simulink model "BSCU_Brake_cmd_tmp"  (Simulink 8.4)
settings: Solver=ode45  StartTime=0.0  StopTime=10.0  RelTol=1e-3
undefined symbols (not defined in the file): BRAKE_PRESSURE_LO, BRAKE_PRESSURE_MAX, BRAKE_PRESSURE_MED, LO, MANUAL, MAX, MED
settings Model: Creator=bourbouh  LastModifiedBy=hbourbou  CovSFcnEnable=on
settings DataIOCC: LimitDataPoints=off  SaveFormat=StructureWithTime  SignalLoggingSaveFormat=Dataset
settings OptimizationCC: ExpressionDepthLimit=128
settings DebuggingCC: UnderspecifiedInitializationDetection=Simplified  MergeDetectMultiDrivingBlocksExec=error  SolverPrmCheckMsg=none  FcnCallInpInsideContextMsg=EnableAllAsError  FrameProcessingCompatibilityMsg=error  StateNameClashWarn=none
settings HardwareCC: ProdBitPerPointer=64  ProdLargestAtomicFloat=Float  ProdIntDivRoundTo=Zero  ProdEndianess=LittleEndian  ProdHWDeviceType=Specified
settings ModelReferenceCC: PropagateSignalLabelsOutOfModel=on
settings GRTTargetCC: CombineOutputUpdateFcns=on  GRTInterface=off

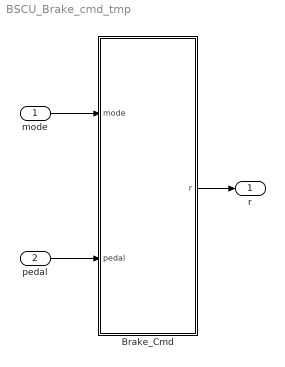
== system BSCU_Brake_cmd_tmp ==
  mode : Inport
  pedal : Inport  Port=2
  Brake_Cmd : Stateflow chart  TreatAsAtomicUnit=on
      settings: PermitHierarchicalResolution=ParametersOnly
  r : Outport
  wires:
  mode/1 -> Brake_Cmd/1(mode)
  pedal/1 -> Brake_Cmd/2(pedal)
  Brake_Cmd/1(r) -> r/1

== stateflow chart Brake_Cmd ==
  (default) -> (junction 13)
  (junction 13) -> (junction 14) [order 1] : [mode == LO]
  (junction 13) -> (junction 15) [order 2]
  (junction 14) -> (junction 23) : {
      | r = BRAKE_PRESSURE_LO;
      | }
  (junction 15) -> (junction 16) [order 1] : [mode == MED ]
  (junction 15) -> (junction 17) [order 2]
  (junction 16) -> (junction 22) : {
      | r = BRAKE_PRESSURE_MED;
      | }
  (junction 17) -> (junction 18) [order 1] : [mode == MAX]
  (junction 17) -> (junction 19) [order 2]
  (junction 18) -> (junction 21) : {
      | r = BRAKE_PRESSURE_MAX;
      | }
  (junction 19) -> (junction 20) : {
      | r = pedal;
      | }
  (junction 21) -> (junction 20)
  (junction 22) -> (junction 21)
  (junction 23) -> (junction 22)
  (junction 20) -> (junction 24)
  data: mode input int32; pedal input int32; r output int32; MANUAL parameter uint8 =1; LO parameter uint8 =2; MED parameter uint8 =3; MAX parameter uint8 =4; BRAKE_PRESSURE_LO parameter double; BRAKE_PRESSURE_MAX parameter double; BRAKE_PRESSURE_MED parameter double
